simulink subsystem "Simulation"  (R2023a)
settings: Solver=VariableStepAuto  StartTime=0.0  StopTime=10.0  RelTol=1e-3
libraries: simulink_extras x3, robotcorelib x1, uavutilslib x1, dspnetwork x1, etargetslib x1
settings Model: Creator=jipva  LastModifiedBy=jipva

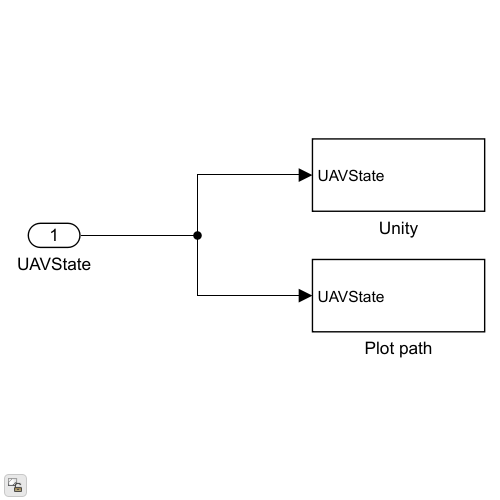
[thumbnail: Simulink's stored preview of the top-level diagram]
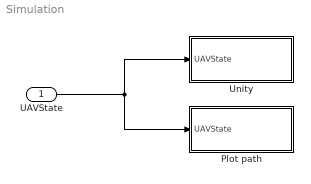
== system Simulation ==
  UAVState : Inport
  Plot path : Subsystem
  Unity : Subsystem
  wires:
  UAVState/1 -> Plot path/1(UAVState), Unity/1(UAVState)

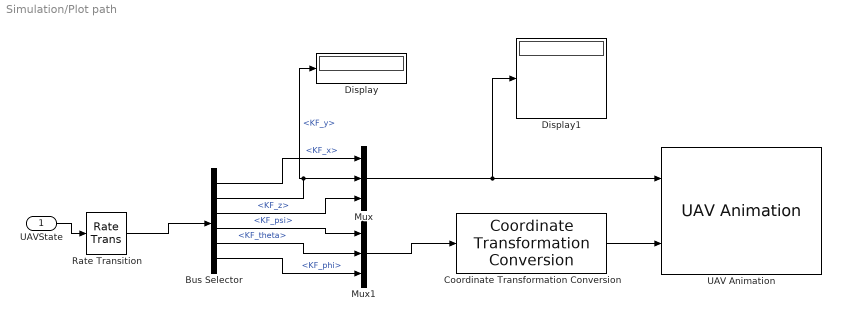
== system Simulation/Plot path ==
  UAVState : Inport
  Bus Selector : BusSelector  OutputSignals=KF_pos.KF_x,KF_pos.KF_y,KF_pos.KF_z,KF_att.KF_psi,KF_att.KF_theta,KF_att.KF_phi
  Coordinate Transformation Conversion : robotcorelib/Coordinate Transformation Conversion  InputRepresentation=Euler Angles  InputEulerSequence=ZYX  ShowTrVecInputPort=on  OutputRepresentation=Quaternion  OutputEulerSequence=ZYX  ShowTrVecOutputPort=on  SimulateUsing=Code generation
      settings: LibrarySourceBlock=navlib/Utilities/Coordinate Transformation Conversion
  Display : Display
  Display1 : Display
  Mux : Mux  Inputs=3
  Mux1 : Mux  Inputs=3
  Rate Transition : RateTransition  OutPortSampleTime=1
  UAV Animation : uavutilslib/UAV Animation  UAVType=Multirotor  UAVSize=1  InertialZDirection=Down  SampleTime=-1
  wires:
  Mux/1 -> UAV Animation/1, Display1/1
  Coordinate Transformation Conversion/1 -> UAV Animation/2
  Mux1/1 -> Coordinate Transformation Conversion/1
  Bus Selector/6 -> Mux1/3  "<KF_phi>"
  Bus Selector/5 -> Mux1/2  "<KF_theta>"
  Bus Selector/4 -> Mux1/1  "<KF_psi>"
  Bus Selector/3 -> Mux/3  "<KF_z>"
  Bus Selector/2 -> Display/1, Mux/2  "<KF_y>"
  Bus Selector/1 -> Mux/1  "<KF_x>"
  Rate Transition/1 -> Bus Selector/1
  UAVState/1 -> Rate Transition/1

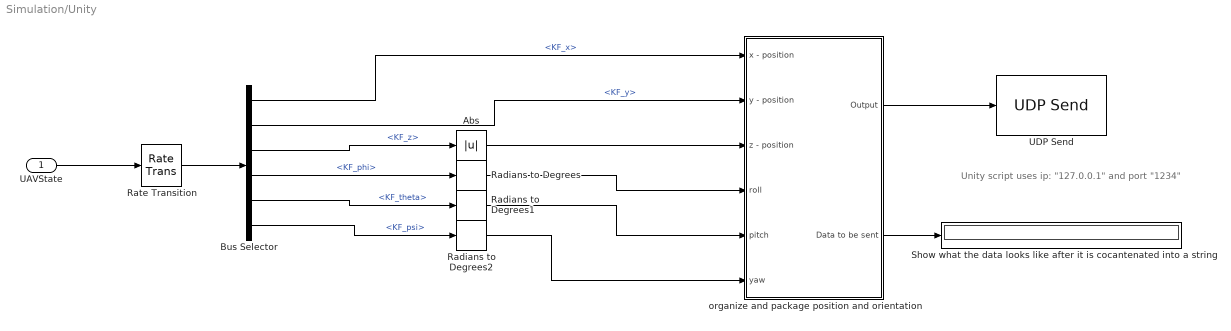
== system Simulation/Unity ==
  note: Unity script uses ip: "127.0.0.1" and port "1234"
  UAVState : Inport
  Abs : Abs  SaturateOnIntegerOverflow=off
  Bus Selector : BusSelector  OutputSignals=KF_pos.KF_x,KF_pos.KF_y,KF_pos.KF_z,KF_att.KF_phi,KF_att.KF_theta,KF_att.KF_psi
  Radians to Degrees : simulink_extras/Transformations/Radians to Degrees
  Radians to Degrees1 : simulink_extras/Transformations/Radians to Degrees
  Radians to Degrees2 : simulink_extras/Transformations/Radians to Degrees
  Rate Transition : RateTransition  OutPortSampleTime=1
  Show what the data looks like after it is cocantenated into a string : Display
  UDP Send : dspnetwork/UDP Send  remoteURL='127.0.0.1'  remotePort=1234  localURL='0.0.0.0'  localPortSource=Automatically determine  localPort=-1  sendBufferSize=8192  sampletime=-1  blockPlatform=HOST  separateLengthPort=0
  organize and package position and orientation : Subsystem
  wires:
  Abs/1 -> organize and package position and orientation/3(z - position)
  Bus Selector/3 -> Abs/1  "<KF_z>"
  Radians to Degrees2/1 -> organize and package position and orientation/6(yaw)
  Radians to Degrees1/1 -> organize and package position and orientation/5(pitch)
  Radians to Degrees/1 -> organize and package position and orientation/4(roll)
  Bus Selector/4 -> Radians to Degrees/1  "<KF_phi>"
  Bus Selector/5 -> Radians to Degrees1/1  "<KF_theta>"
  Bus Selector/6 -> Radians to Degrees2/1  "<KF_psi>"
  Bus Selector/2 -> organize and package position and orientation/2(y - position)  "<KF_y>"
  Bus Selector/1 -> organize and package position and orientation/1(x - position)  "<KF_x>"
  Rate Transition/1 -> Bus Selector/1
  UAVState/1 -> Rate Transition/1
  organize and package position and orientation/2(Data to be sent) -> Show what the data looks like after it is cocantenated into a string/1
  organize and package position and orientation/1(Output) -> UDP Send/1

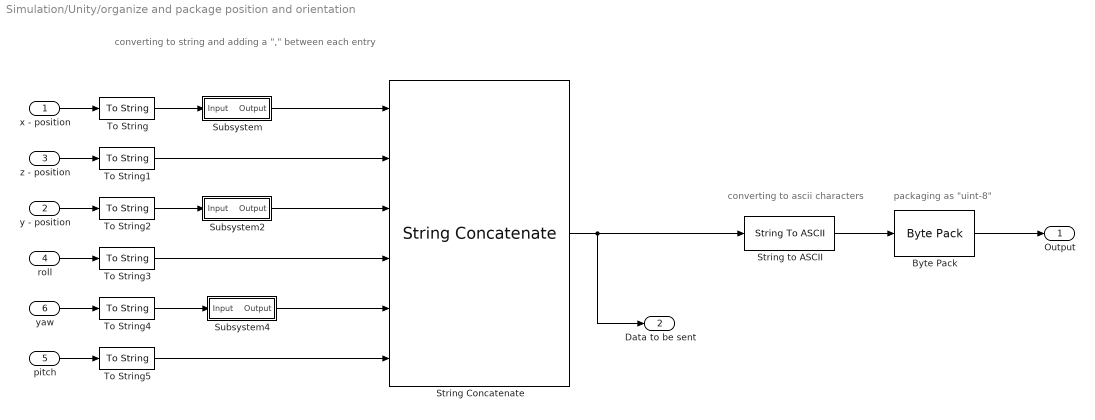
== system Simulation/Unity/organize and package position and orientation ==
  note: converting to string and adding a "," between each entry
  note: converting to ascii characters
  note: packaging as "uint-8"
  x - position : Inport
  y - position : Inport  Port=2
  z - position : Inport  Port=3
  roll : Inport  Port=4
  pitch : Inport  Port=5
  yaw : Inport  Port=6
  Byte Pack : etargetslib/Byte Pack  datatypes={'uint8'}  byteAlign=1
  String Concatenate : StringConcatenate  Inputs=6
  String to ASCII : StringToASCII  OutputVectorSize=64
  Subsystem : Subsystem
  Subsystem2 : Subsystem
  Subsystem4 : Subsystem
  To String{,1..5} (6 alike) : ToString
  Output : Outport
  Data to be sent : Outport  Port=2
  wires:
  y - position/1 -> To String2/1
  yaw/1 -> To String4/1
  roll/1 -> To String3/1
  pitch/1 -> To String5/1
  x - position/1 -> To String/1
  z - position/1 -> To String1/1
  Byte Pack/1 -> Output/1
  Subsystem/1(Output) -> String Concatenate/1
  To String4/1 -> Subsystem4/1(Input)
  To String1/1 -> String Concatenate/2
  Subsystem2/1(Output) -> String Concatenate/3
  To String5/1 -> String Concatenate/6
  To String/1 -> Subsystem/1(Input)
  String to ASCII/1 -> Byte Pack/1
  Subsystem4/1(Output) -> String Concatenate/5
  To String2/1 -> Subsystem2/1(Input)
  To String3/1 -> String Concatenate/4
  String Concatenate/1 -> String to ASCII/1, Data to be sent/1

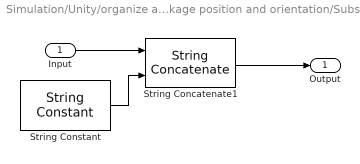
== system Simulation/Unity/organize and package position and orientation/Subsystem ==
  Input : Inport
  String Concatenate1 : StringConcatenate
  String Constant : StringConstant  String="\",\""
  Output : Outport
  wires:
  String Concatenate1/1 -> Output/1
  String Constant/1 -> String Concatenate1/2
  Input/1 -> String Concatenate1/1

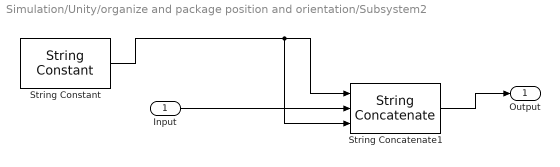
== system Simulation/Unity/organize and package position and orientation/Subsystem2 ==
  Input : Inport
  String Concatenate1 : StringConcatenate  Inputs=3
  String Constant : StringConstant  String="\",\""
  Output : Outport
  wires:
  String Constant/1 -> String Concatenate1/1, String Concatenate1/3
  Input/1 -> String Concatenate1/2
  String Concatenate1/1 -> Output/1

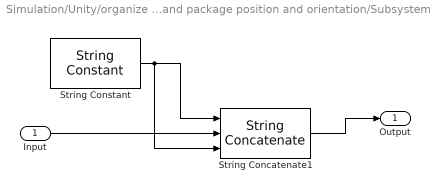
== system Simulation/Unity/organize and package position and orientation/Subsystem4 ==
  Input : Inport
  String Concatenate1 : StringConcatenate  Inputs=3
  String Constant : StringConstant  String="\",\""
  Output : Outport
  wires:
  String Constant/1 -> String Concatenate1/1, String Concatenate1/3
  Input/1 -> String Concatenate1/2
  String Concatenate1/1 -> Output/1
